simulink model "hespanha1"  (R2020a)
settings: Solver=FixedStepAuto  StartTime=0.0  StopTime=50  FixedStep=0.001  RelTol=1e-3
values from neighbouring files (symbols this model uses):
  ss1 = ss(K1)    [lpv_config.m]
  sysP = ss(P)    [lpv_config.m]
undefined symbols (not defined in the file or in its folder): options
libraries: simulink x2
settings Model: Creator=kekatos  LastModifiedBy=kekatos
settings DataIOCC: SignalLogging=off  DSMLogging=off  ReturnWorkspaceOutputs=off

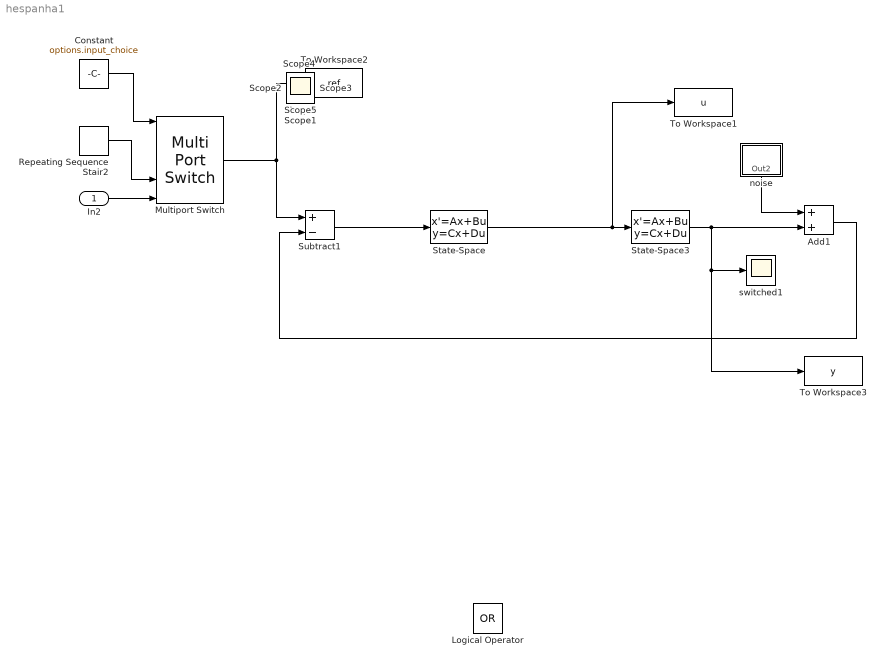
== system hespanha1 ==
  In2 : Inport
  Add1 : Sum
  Constant : Constant  Value=options.input_choice
  Logical Operator : Logic  Operator=OR  AllPortsSameDT=off  OutDataTypeStr=boolean
  Multiport Switch : MultiPortSwitch  Inputs=4
  Repeating Sequence Stair2 : simulink/Sources/Repeating Sequence Stair  OutValues=options.sim_cov  tsamp=options.ref_Ts  OutMin=[]  OutMax=[]  OutDataTypeStr=double  OutputDataTypeScalingMode=double  OutDataType=fixdt(0,8)  ConRadixGroup=Best Precision: Vector-wise  OutScaling=2^-12
  State-Space : StateSpace  A=ss1.A  B=ss1.B  C=ss1.C  D=ss1.D  InitialCondition=0
  State-Space3 : StateSpace  A=sysP.A  B=sysP.B  C=sysP.C  D=sysP.D  InitialCondition=0
  Subtract1 : Sum  Inputs=+-
  To Workspace1 : ToWorkspace  VariableName=u  SaveFormat=Structure With Time  SampleTime=options.dt
  To Workspace2 : ToWorkspace  VariableName=ref  SaveFormat=Structure With Time  SampleTime=options.dt
  To Workspace3 : ToWorkspace  VariableName=y  SaveFormat=Structure With Time  SampleTime=options.dt
  noise : Subsystem
  switched1 : Scope
  Scope{,1..5} (6 alike) : Scope
  wires:
  State-Space/1 -> State-Space3/1, To Workspace1/1
  Multiport Switch/1 -> Subtract1/1, To Workspace2/1
  Add1/1 -> Subtract1/2
  State-Space3/1 -> switched1/1, To Workspace3/1, Add1/2
  Subtract1/1 -> State-Space/1
  Constant/1 -> Multiport Switch/1
  Repeating Sequence Stair2/1 -> Multiport Switch/4
  In2/1 -> Multiport Switch/5
  noise/1(Out2) -> Add1/1

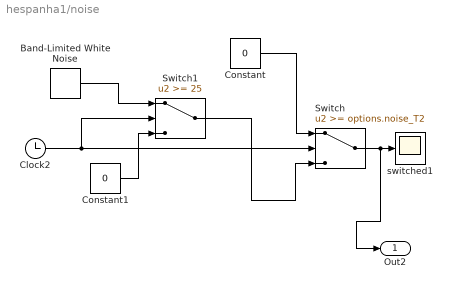
== system hespanha1/noise ==
  Band-Limited White Noise : simulink/Sources/Band-Limited White Noise  Cov=1e-6  Ts=options.dt  seed=randi(1000)
  Clock2 : Clock
  Constant : Constant  Value=0
  Constant1 : Constant  Value=0
  Switch : Switch  Threshold=options.noise_T2
  Switch1 : Switch  Threshold=25
  switched1 : Scope
  Out2 : Outport
  wires:
  Clock2/1 -> Switch1/2, Switch/2
  Constant/1 -> Switch/1
  Constant1/1 -> Switch1/3
  Band-Limited White Noise/1 -> Switch1/1
  Switch/1 -> Out2/1, switched1/1
  Switch1/1 -> Switch/3
